simulink model "FlightGear_PID_try"  (R2017a)
settings: Solver=VariableStepAuto  StartTime=0.0  StopTime=20  RelTol=1e-3
values from neighbouring files (symbols this model uses):
  Fext_N = -g_EN * m    [HW5_4_surfaces.m]    (also in TEST_aerosetup.m = [10 10 10]; surfaces_setup_test.m)
  g_EN = [0; 0; 9.81]    [HW5_4_surfaces.m]    (also in TEST_aerosetup.m = [0; 0; 9.8]; surfaces_setup_test.m)
  J_cg = ones(3)    [HW5_4_surfaces.m]    (also in TEST_aerosetup.m)
  M_total = sum(MnG(:,1))/1000    [HW5_4_surfaces.m]    (also in TEST_aerosetup.m; surfaces_setup_test.m = sum(MnG1(:,1))/1000)
  Mext_B = [0; 0; 0]    [HW5_4_surfaces.m]    (also in TEST_aerosetup.m = [1; 1; 1]; surfaces_setup_test.m)
  p_E_BE_ini = p_E_BE_ini_deg .* [deg2rad; deg2rad; 1]    [HW5_4_surfaces.m]    (also in TEST_aerosetup.m; surfaces_setup_test.m)
  Rearth = 6371000    [HW5_4_surfaces.m]    (also in TEST_aerosetup.m; surfaces_setup_test.m)
  Theta_ini = Theta_ini_deg * deg2rad    [HW5_4_surfaces.m]    (also in TEST_aerosetup.m; surfaces_setup_test.m)
  v_N_AE = [0;0;0]    [HW5_4_surfaces.m]    (also in TEST_aerosetup.m; surfaces_setup_test.m)
  Vbbe_int = [10; 0; 0]    [HW5_4_surfaces.m]    (also in TEST_aerosetup.m; surfaces_setup_test.m = [5; 0; 0])
  w_B_BE_ini = [1e0; 1e-2; 1e-2]    [HW5_4_surfaces.m]    (also in TEST_aerosetup.m; surfaces_setup_test.m)
undefined symbols (not defined in the file or in its folder): Earth, WGS84
libraries: simulink x4, dspinverses x3, aerolibfltsims x2, vrlib x2, sharedtransform x1, aerolibtransform2 x1
settings Model: Creator=Jiaoran Wang  LastModifiedBy=Jiaoran Wang

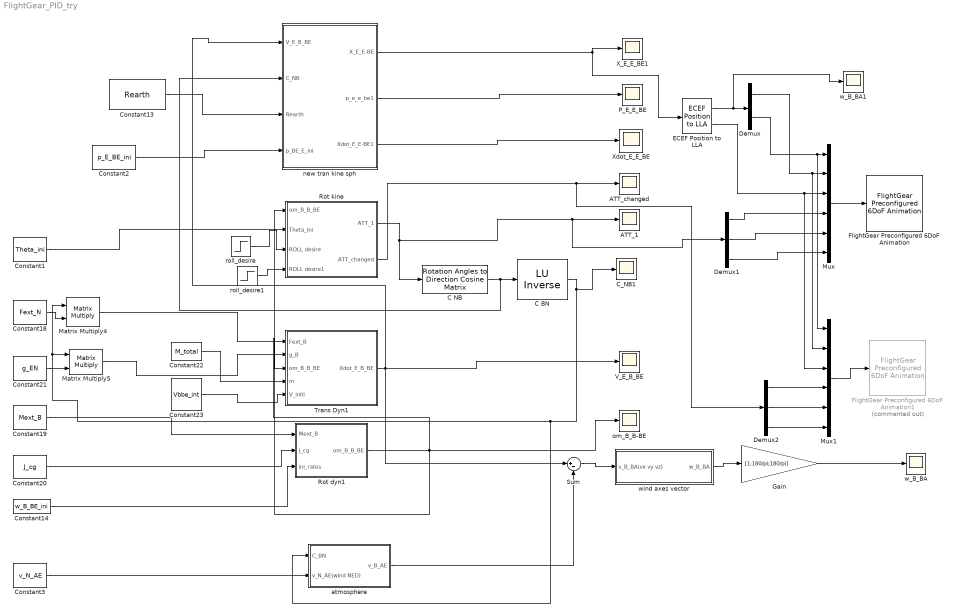
== system FlightGear_PID_try ==
  ATT_1 : Scope
  ATT_changed : Scope
  C BN : dspinverses/ LU Inverse
      settings: SourceProductName=DSP System Toolbox
  C NB : sharedtransform/Rotation Angles to Direction Cosine Matrix  rotationOrder=ZYX
  C_NB1 : Scope
  Constant1 : Constant  Value=Theta_ini
  Constant13 : Constant  Value=Rearth
  Constant14 : Constant  Value=w_B_BE_ini
  Constant18 : Constant  Value=Fext_N
  Constant19 : Constant  Value=Mext_B
  Constant2 : Constant  Value=p_E_BE_ini  VectorParams1D=off
  Constant20 : Constant  Value=J_cg
  Constant21 : Constant  Value=g_EN
  Constant22 : Constant  Value=M_total
  Constant23 : Constant  Value=Vbbe_int
  Constant3 : Constant  Value=v_N_AE
  Demux : Demux  Outputs=2
  Demux1 : Demux  Outputs=3
  Demux2 : Demux  Outputs=3
  ECEF Position to LLA : aerolibtransform2/ECEF Position to LLA  units=Metric (MKS)  ptype=Earth (WGS84)  F=1/298.257223563  R=6378137
      settings: SourceProductName=Aerospace Blockset  SourceProductBaseCode=AE
  FlightGear Preconfigured 6DoF Animation : aerolibfltsims/FlightGear Preconfigured 6DoF Animation  xFlightGearVersion=v3.0  DestinationIpAddress=127.0.0.1  DestinationPort=5502  SampleTime=1/50
      settings: SourceProductName=Aerospace Blockset
  FlightGear Preconfigured 6DoF Animation1 : aerolibfltsims/FlightGear Preconfigured 6DoF Animation  Commented=on  xFlightGearVersion=v3.0  DestinationIpAddress=127.0.0.1  DestinationPort=5502  SampleTime=1/50
      settings: SourceProductName=Aerospace Blockset
  Gain : Gain  Gain=[1;180/pi;180/pi]
  Matrix Multiply4 : Product  Multiplication=Matrix(*)
  Matrix Multiply5 : Product  Multiplication=Matrix(*)
  Mux : Mux  Inputs=6
  Mux1 : Mux  Inputs=6
  P_E_E_BE : Scope
  Rot dyn1 : Subsystem
  Rot kine : Subsystem
  Sum : Sum  Inputs=|+-
  Trans Dyn1 : Subsystem
  V_E_B_BE : Scope
  "X_E_E_BE1 " : Scope
  Xdot_E_E_BE : Scope
  atmosphere : Subsystem
  new tran kine sph : Subsystem
  om_B_B-BE : Scope
  roll_desire : Step  Time=0  After=0  SampleTime=0
  roll_desire1 : Step  Time=0  After=0  SampleTime=0
  w_B_BA : Scope
  w_B_BA1 : Scope
  wind axes vector : Subsystem
  wires:
  ECEF Position to LLA/1 -> w_B_BA1/1, Demux/1
  Constant2/1 -> new tran kine sph/4(p_BE_E_ini)
  Constant13/1 -> new tran kine sph/3(Rearth)
  C BN/1 -> C_NB1/1, atmosphere/1(C_BN), Matrix Multiply5/1, Matrix Multiply4/1
  Matrix Multiply5/1 -> Trans Dyn1/2(g_B)
  Demux/1 -> Mux1/2, Mux/2
  new tran kine sph/2(p_e_e_be1) -> P_E_E_BE/1
  Constant23/1 -> Trans Dyn1/5(V_initi)
  Matrix Multiply4/1 -> Trans Dyn1/1(Fext_B)
  Demux1/2 -> Mux/5
  ECEF Position to LLA/2 -> Mux1/3, Mux/3
  Constant18/1 -> Matrix Multiply4/2
  wind axes vector/1(w_B_BA) -> Gain/1
  atmosphere/1(v_B_AE) -> Sum/2
  Demux/2 -> Mux1/1, Mux/1
  Constant19/1 -> Rot dyn1/1(Mext_B)
  Constant3/1 -> atmosphere/2(v_N_AE(wind NED))
  new tran kine sph/1(X_E_E-BE) -> "X_E_E_BE1 "/1, ECEF Position to LLA/1
  new tran kine sph/3(Xdot_E_E-BE1) -> Xdot_E_E_BE/1
  Rot dyn1/1(om_B_B_BE) -> Rot kine/1(om_B_B_BE), om_B_B-BE/1, Trans Dyn1/3(om_B_B_BE)
  Constant14/1 -> Rot dyn1/3(ini_rates)
  Constant1/1 -> Rot kine/2(Theta_ini)
  Trans Dyn1/1(Xdot_E_B_BE) -> V_E_B_BE/1, Sum/1, new tran kine sph/1(V_E_B_BE)
  Constant22/1 -> Trans Dyn1/4(m)
  Constant21/1 -> Matrix Multiply5/2
  C NB/1 -> new tran kine sph/2(C_NB), C BN/1
  Sum/1 -> wind axes vector/1(v_B_BA(vx vy vz))
  Rot kine/1(ATT_1) -> Demux1/1, ATT_1/1, C NB/1
  Constant20/1 -> Rot dyn1/2(J_cg)
  Demux1/1 -> Mux/4
  Mux/1 -> FlightGear Preconfigured 6DoF Animation/1
  Gain/1 -> w_B_BA/1
  Demux1/3 -> Mux/6
  Rot kine/2(ATT_changed) -> Demux2/1, ATT_changed/1
  roll_desire/1 -> Rot kine/3(ROLL desire)
  roll_desire1/1 -> Rot kine/4(ROLL desire1)
  Mux1/1 -> FlightGear Preconfigured 6DoF Animation1/1
  Demux2/3 -> Mux1/6
  Demux2/2 -> Mux1/5
  Demux2/1 -> Mux1/4

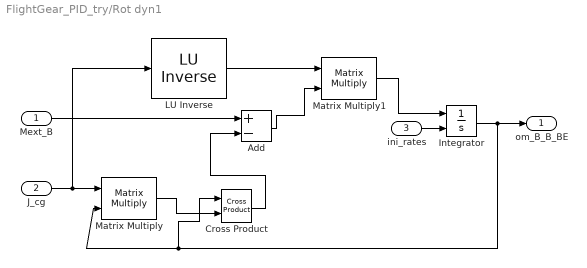
== system FlightGear_PID_try/Rot dyn1 ==
  Mext_B : Inport
  J_cg : Inport  Port=2
  ini_rates : Inport  Port=3
  " LU Inverse" : dspinverses/ LU Inverse
      settings: SourceProductName=DSP System Toolbox
  Add : Sum  Inputs=+-
  Cross Product : vrlib/Utilities/Cross Product
      settings: SourceProductBaseCode=VR
  Integrator : Integrator  InitialConditionSource=external
  Matrix Multiply : Product  Multiplication=Matrix(*)
  Matrix Multiply1 : Product  Multiplication=Matrix(*)
  om_B_B_BE : Outport
  wires:
  Mext_B/1 -> Add/1
  J_cg/1 -> " LU Inverse"/1, Matrix Multiply/1
  Matrix Multiply/1 -> Cross Product/2
  " LU Inverse"/1 -> Matrix Multiply1/1
  Add/1 -> Matrix Multiply1/2
  Cross Product/1 -> Add/2
  Matrix Multiply1/1 -> Integrator/1
  ini_rates/1 -> Integrator/2
  Integrator/1 -> Cross Product/1, Matrix Multiply/2, om_B_B_BE/1

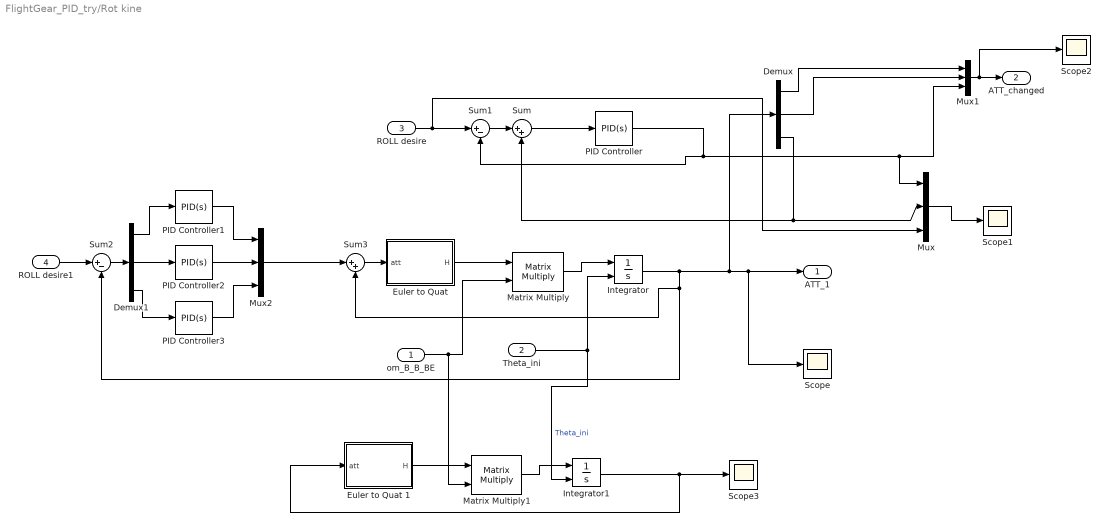
== system FlightGear_PID_try/Rot kine ==
  om_B_B_BE : Inport
  Theta_ini : Inport  Port=2
  ROLL desire : Inport  Port=3
  ROLL desire1 : Inport  Port=4
  Demux : Demux  Outputs=3
  Demux1 : Demux  Outputs=3
  "Euler to Quat " : MATLAB Function  TreatAsAtomicUnit=on
  Euler to Quat 1 : MATLAB Function  TreatAsAtomicUnit=on
  Integrator : Integrator  InitialConditionSource=external
  Integrator1 : Integrator  InitialConditionSource=external
  Matrix Multiply : Product  Multiplication=Matrix(*)
  Matrix Multiply1 : Product  Multiplication=Matrix(*)
  Mux : Mux  Inputs=3
  Mux1 : Mux  Inputs=3
  Mux2 : Mux  Inputs=3
  PID Controller : simulink/Continuous/PID Controller  Controller=PID  TimeDomain=Continuous-time  SampleTime=-1  IntegratorMethod=Forward Euler  FilterMethod=Forward Euler  Form=Parallel  UseFilter=on  ControllerParametersSource=internal  P=0  I=10  D=0  N=100  InitialConditionSource=internal  InitialConditionForIntegrator=0  InitialConditionForFilter=0  ExternalReset=none  LimitOutput=off  UpperSaturationLimit=inf  LowerSaturationLimit=-inf  LinearizeAsGain=on  AntiWindupMode=none  Kb=1  TrackingMode=off  Kt=1  PParamMin=[]  PParamMax=[]  IParamMin=[]  IParamMax=[]  DParamMin=[]  DParamMax=[]  NParamMin=[]  NParamMax=[]  KbParamMin=[]  KbParamMax=[]  KtParamMin=[]  KtParamMax=[]  POutMin=[]  POutMax=[]  IOutMin=[]  IOutMax=[]  DOutMin=[]  DOutMax=[]  NOutMin=[]  NOutMax=[]  KbOutMin=[]  KbOutMax=[]  KtOutMin=[]  KtOutMax=[]  IntegratorOutMin=[]  IntegratorOutMax=[]  FilterOutMin=[]  FilterOutMax=[]  SumOutMin=[]  SumOutMax=[]  SumI1OutMin=[]  SumI1OutMax=[]  SumI2OutMin=[]  SumI2OutMax=[]  SumI3OutMin=[]  SumI3OutMax=[]  SumDOutMin=[]  SumDOutMax=[]  SaturationOutMin=[]  SaturationOutMax=[]  IntegratorContinuousStateAttributes=''  IntegratorStateMustResolveToSignalObject=off  IntegratorRTWStateStorageClass=Auto  FilterContinuousStateAttributes=''  FilterStateMustResolveToSignalObject=off  FilterRTWStateStorageClass=Auto  DifferentiatorICPrevScaledInput=0  DifferentiatorOutMin=[]  DifferentiatorOutMax=[]  InitialConditionSetting=State (most efficient)
  PID Controller1 : simulink/Continuous/PID Controller  Controller=PID  TimeDomain=Continuous-time  SampleTime=-1  IntegratorMethod=Forward Euler  FilterMethod=Forward Euler  Form=Parallel  UseFilter=on  ControllerParametersSource=internal  P=0  I=10  D=1  N=100  InitialConditionSource=internal  InitialConditionForIntegrator=0  InitialConditionForFilter=0  ExternalReset=none  LimitOutput=off  UpperSaturationLimit=inf  LowerSaturationLimit=-inf  LinearizeAsGain=on  AntiWindupMode=none  Kb=1  TrackingMode=off  Kt=1  PParamMin=[]  PParamMax=[]  IParamMin=[]  IParamMax=[]  DParamMin=[]  DParamMax=[]  NParamMin=[]  NParamMax=[]  KbParamMin=[]  KbParamMax=[]  KtParamMin=[]  KtParamMax=[]  POutMin=[]  POutMax=[]  IOutMin=[]  IOutMax=[]  DOutMin=[]  DOutMax=[]  NOutMin=[]  NOutMax=[]  KbOutMin=[]  KbOutMax=[]  KtOutMin=[]  KtOutMax=[]  IntegratorOutMin=[]  IntegratorOutMax=[]  FilterOutMin=[]  FilterOutMax=[]  SumOutMin=[]  SumOutMax=[]  SumI1OutMin=[]  SumI1OutMax=[]  SumI2OutMin=[]  SumI2OutMax=[]  SumI3OutMin=[]  SumI3OutMax=[]  SumDOutMin=[]  SumDOutMax=[]  SaturationOutMin=[]  SaturationOutMax=[]  IntegratorContinuousStateAttributes=''  IntegratorStateMustResolveToSignalObject=off  IntegratorRTWStateStorageClass=Auto  FilterContinuousStateAttributes=''  FilterStateMustResolveToSignalObject=off  FilterRTWStateStorageClass=Auto  DifferentiatorICPrevScaledInput=0  DifferentiatorOutMin=[]  DifferentiatorOutMax=[]  InitialConditionSetting=State (most efficient)
  PID Controller2 : simulink/Continuous/PID Controller  Controller=PID  TimeDomain=Continuous-time  SampleTime=-1  IntegratorMethod=Forward Euler  FilterMethod=Forward Euler  Form=Parallel  UseFilter=on  ControllerParametersSource=internal  P=0  I=10  D=0  N=100  InitialConditionSource=internal  InitialConditionForIntegrator=0  InitialConditionForFilter=0  ExternalReset=none  LimitOutput=off  UpperSaturationLimit=inf  LowerSaturationLimit=-inf  LinearizeAsGain=on  AntiWindupMode=none  Kb=1  TrackingMode=off  Kt=1  PParamMin=[]  PParamMax=[]  IParamMin=[]  IParamMax=[]  DParamMin=[]  DParamMax=[]  NParamMin=[]  NParamMax=[]  KbParamMin=[]  KbParamMax=[]  KtParamMin=[]  KtParamMax=[]  POutMin=[]  POutMax=[]  IOutMin=[]  IOutMax=[]  DOutMin=[]  DOutMax=[]  NOutMin=[]  NOutMax=[]  KbOutMin=[]  KbOutMax=[]  KtOutMin=[]  KtOutMax=[]  IntegratorOutMin=[]  IntegratorOutMax=[]  FilterOutMin=[]  FilterOutMax=[]  SumOutMin=[]  SumOutMax=[]  SumI1OutMin=[]  SumI1OutMax=[]  SumI2OutMin=[]  SumI2OutMax=[]  SumI3OutMin=[]  SumI3OutMax=[]  SumDOutMin=[]  SumDOutMax=[]  SaturationOutMin=[]  SaturationOutMax=[]  IntegratorContinuousStateAttributes=''  IntegratorStateMustResolveToSignalObject=off  IntegratorRTWStateStorageClass=Auto  FilterContinuousStateAttributes=''  FilterStateMustResolveToSignalObject=off  FilterRTWStateStorageClass=Auto  DifferentiatorICPrevScaledInput=0  DifferentiatorOutMin=[]  DifferentiatorOutMax=[]  InitialConditionSetting=State (most efficient)
  PID Controller3 : simulink/Continuous/PID Controller  Controller=PID  TimeDomain=Continuous-time  SampleTime=-1  IntegratorMethod=Forward Euler  FilterMethod=Forward Euler  Form=Parallel  UseFilter=on  ControllerParametersSource=internal  P=0  I=10  D=0  N=100  InitialConditionSource=internal  InitialConditionForIntegrator=0  InitialConditionForFilter=0  ExternalReset=none  LimitOutput=off  UpperSaturationLimit=inf  LowerSaturationLimit=-inf  LinearizeAsGain=on  AntiWindupMode=none  Kb=1  TrackingMode=off  Kt=1  PParamMin=[]  PParamMax=[]  IParamMin=[]  IParamMax=[]  DParamMin=[]  DParamMax=[]  NParamMin=[]  NParamMax=[]  KbParamMin=[]  KbParamMax=[]  KtParamMin=[]  KtParamMax=[]  POutMin=[]  POutMax=[]  IOutMin=[]  IOutMax=[]  DOutMin=[]  DOutMax=[]  NOutMin=[]  NOutMax=[]  KbOutMin=[]  KbOutMax=[]  KtOutMin=[]  KtOutMax=[]  IntegratorOutMin=[]  IntegratorOutMax=[]  FilterOutMin=[]  FilterOutMax=[]  SumOutMin=[]  SumOutMax=[]  SumI1OutMin=[]  SumI1OutMax=[]  SumI2OutMin=[]  SumI2OutMax=[]  SumI3OutMin=[]  SumI3OutMax=[]  SumDOutMin=[]  SumDOutMax=[]  SaturationOutMin=[]  SaturationOutMax=[]  IntegratorContinuousStateAttributes=''  IntegratorStateMustResolveToSignalObject=off  IntegratorRTWStateStorageClass=Auto  FilterContinuousStateAttributes=''  FilterStateMustResolveToSignalObject=off  FilterRTWStateStorageClass=Auto  DifferentiatorICPrevScaledInput=0  DifferentiatorOutMin=[]  DifferentiatorOutMax=[]  InitialConditionSetting=State (most efficient)
  Scope{,1..3} (4 alike) : Scope
  Sum : Sum  Inputs=|++
  Sum1 : Sum  Inputs=|+-
  Sum2 : Sum  Inputs=|+-
  Sum3 : Sum  Inputs=|++
  ATT_1 : Outport
  ATT_changed : Outport  Port=2
  wires:
  om_B_B_BE/1 -> Matrix Multiply1/2, Matrix Multiply/2
  Integrator/1 -> Sum3/2, Sum2/2, Scope/1, ATT_1/1, Demux/1
  "Euler to Quat "/1(H) -> Matrix Multiply/1
  Theta_ini/1 -> Integrator/2, Integrator1/2  "Theta_ini"
  Matrix Multiply/1 -> Integrator/1
  Demux/3 -> Sum/2, Mux/2
  Demux/1 -> Mux1/1
  PID Controller/1 -> Sum1/2, Mux/1, Mux1/3
  Mux/1 -> Scope1/1
  Demux/2 -> Mux1/2
  Mux1/1 -> Scope2/1, ATT_changed/1
  ROLL desire/1 -> Sum1/1, Mux/3
  Sum1/1 -> Sum/1
  Sum/1 -> PID Controller/1
  ROLL desire1/1 -> Sum2/1
  Sum3/1 -> "Euler to Quat "/1(att)
  Matrix Multiply1/1 -> Integrator1/1
  Euler to Quat 1/1(H) -> Matrix Multiply1/1
  Demux1/1 -> PID Controller1/1
  Sum2/1 -> Demux1/1
  Demux1/2 -> PID Controller2/1
  Demux1/3 -> PID Controller3/1
  Mux2/1 -> Sum3/1
  PID Controller1/1 -> Mux2/1
  PID Controller2/1 -> Mux2/2
  PID Controller3/1 -> Mux2/3
  Integrator1/1 -> Euler to Quat 1/1(att), Scope3/1

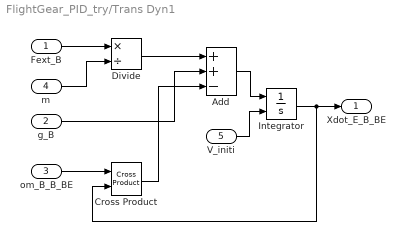
== system FlightGear_PID_try/Trans Dyn1 ==
  Fext_B : Inport
  g_B : Inport  Port=2
  om_B_B_BE : Inport  Port=3
  m : Inport  Port=4
  V_initi : Inport  Port=5
  Add : Sum  Inputs=++-
  Cross Product : vrlib/Utilities/Cross Product
      settings: SourceProductBaseCode=VR
  Divide : Product  Inputs=*/
  Integrator : Integrator  InitialConditionSource=external
  Xdot_E_B_BE : Outport
  wires:
  Fext_B/1 -> Divide/1
  m/1 -> Divide/2
  Divide/1 -> Add/1
  g_B/1 -> Add/2
  om_B_B_BE/1 -> Cross Product/1
  Cross Product/1 -> Add/3
  Add/1 -> Integrator/1
  V_initi/1 -> Integrator/2
  Integrator/1 -> Cross Product/2, Xdot_E_B_BE/1

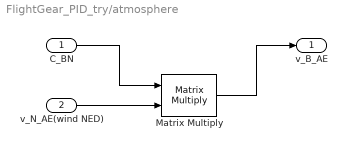
== system FlightGear_PID_try/atmosphere ==
  C_BN : Inport
  v_N_AE(wind NED) : Inport  Port=2
  Matrix Multiply : Product  Multiplication=Matrix(*)
  v_B_AE : Outport
  wires:
  v_N_AE(wind NED)/1 -> Matrix Multiply/2
  C_BN/1 -> Matrix Multiply/1
  Matrix Multiply/1 -> v_B_AE/1

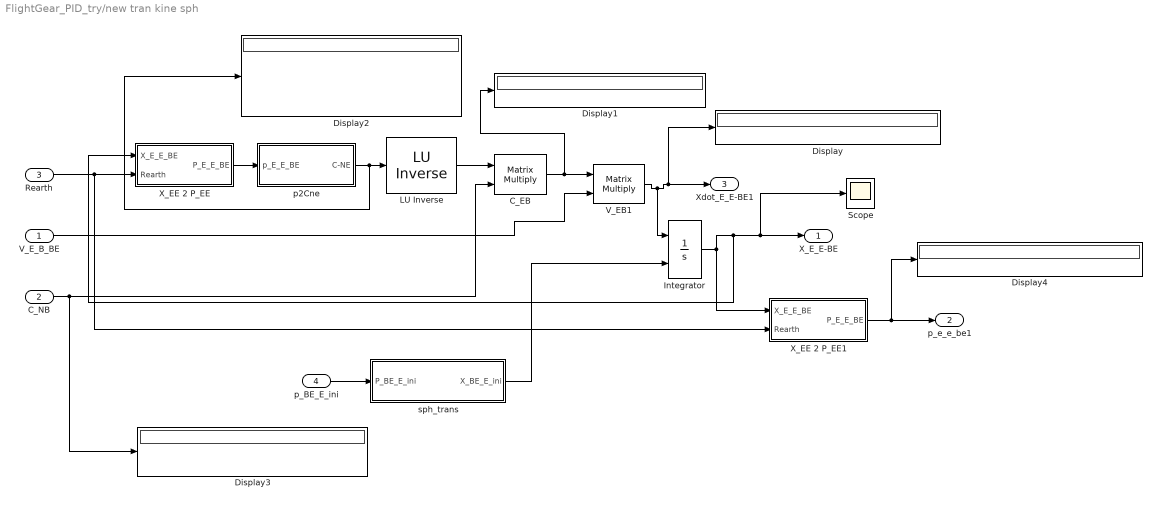
== system FlightGear_PID_try/new tran kine sph ==
  V_E_B_BE : Inport
  C_NB : Inport  Port=2
  Rearth : Inport  Port=3
  p_BE_E_ini : Inport  Port=4
  " LU Inverse" : dspinverses/ LU Inverse
      settings: SourceProductName=DSP System Toolbox
  C_EB : Product  Multiplication=Matrix(*)
  Display{,1..4} (5 alike) : Display
  Integrator : Integrator  InitialConditionSource=external
  Scope : Scope
  V_EB1 : Product  Multiplication=Matrix(*)
  X_EE 2 P_EE : Subsystem
  X_EE 2 P_EE1 : Subsystem
  p2Cne : Subsystem
  sph_trans : MATLAB Function  TreatAsAtomicUnit=on
  X_E_E-BE : Outport
  p_e_e_be1 : Outport  Port=2
  Xdot_E_E-BE1 : Outport  Port=3
  wires:
  " LU Inverse"/1 -> C_EB/1
  Integrator/1 -> Scope/1, X_E_E-BE/1, X_EE 2 P_EE/1(X_E_E_BE), X_EE 2 P_EE1/1(X_E_E_BE)
  X_EE 2 P_EE1/1(P_E_E_BE) -> Display4/1, p_e_e_be1/1
  Rearth/1 -> X_EE 2 P_EE1/2(Rearth), X_EE 2 P_EE/2(Rearth)
  V_EB1/1 -> Display/1, Xdot_E_E-BE1/1, Integrator/1
  C_EB/1 -> Display1/1, V_EB1/1
  p2Cne/1(C-NE) -> Display2/1, " LU Inverse"/1
  X_EE 2 P_EE/1(P_E_E_BE) -> p2Cne/1(p_E_E_BE)
  C_NB/1 -> Display3/1, C_EB/2
  V_E_B_BE/1 -> V_EB1/2
  p_BE_E_ini/1 -> sph_trans/1(P_BE_E_ini)
  sph_trans/1(X_BE_E_ini) -> Integrator/2

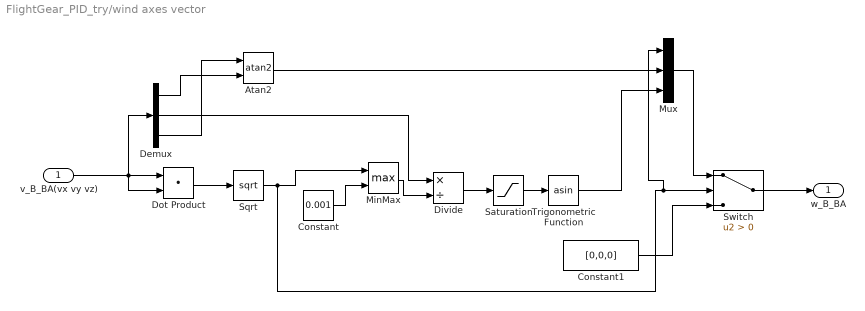
== system FlightGear_PID_try/wind axes vector ==
  v_B_BA(vx vy vz) : Inport
  Atan2 : Trigonometry  Operator=atan2
  Constant : Constant  Value=0.001
  Constant1 : Constant  Value=[0,0,0]
  Demux : Demux  Outputs=3
  Divide : Product  Inputs=*/
  Dot Product : DotProduct  InputSameDT=on  OutDataTypeStr=Inherit: Inherit via internal rule
  MinMax : MinMax  Function=max  Inputs=2
  Mux : Mux  Inputs=3
  Saturation : Saturate
  Sqrt : Sqrt  SaturateOnIntegerOverflow=on
  Switch : Switch  Criteria=u2 > Threshold
  Trigonometric Function : Trigonometry  Operator=asin  ApproximationMethod=CORDIC
  w_B_BA : Outport
  wires:
  v_B_BA(vx vy vz)/1 -> Demux/1, Dot Product/2, Dot Product/1
  Dot Product/1 -> Sqrt/1
  Sqrt/1 -> Mux/1, Switch/2, MinMax/1
  Constant/1 -> MinMax/2
  MinMax/1 -> Divide/2
  Demux/2 -> Divide/1
  Demux/3 -> Atan2/1
  Demux/1 -> Atan2/2
  Atan2/1 -> Mux/2
  Divide/1 -> Saturation/1
  Saturation/1 -> Trigonometric Function/1
  Trigonometric Function/1 -> Mux/3
  Constant1/1 -> Switch/3
  Mux/1 -> Switch/1
  Switch/1 -> w_B_BA/1

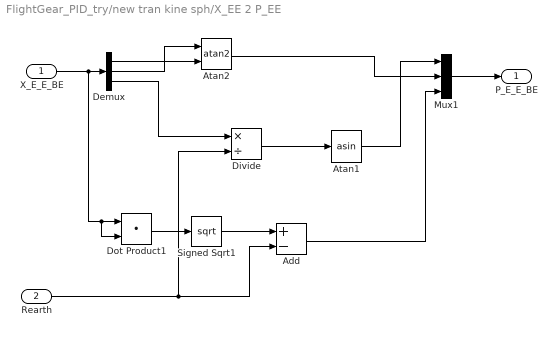
== system FlightGear_PID_try/new tran kine sph/X_EE 2 P_EE ==
  X_E_E_BE : Inport
  Rearth : Inport  Port=2
  Add : Sum  Inputs=+-
  Atan1 : Trigonometry  Operator=asin
  Atan2 : Trigonometry  Operator=atan2
  Demux : Demux  Outputs=3
  Divide : Product  Inputs=*/
  Dot Product1 : DotProduct  InputSameDT=on  OutDataTypeStr=Inherit: Inherit via internal rule
  Mux1 : Mux  Inputs=3
  Signed Sqrt1 : Sqrt  SaturateOnIntegerOverflow=on
  P_E_E_BE : Outport
  wires:
  X_E_E_BE/1 -> Dot Product1/2, Dot Product1/1, Demux/1
  Demux/1 -> Atan2/2
  Demux/2 -> Atan2/1
  Atan2/1 -> Mux1/2
  Dot Product1/1 -> Signed Sqrt1/1
  Signed Sqrt1/1 -> Add/1
  Rearth/1 -> Divide/2, Add/2
  Add/1 -> Mux1/3
  Mux1/1 -> P_E_E_BE/1
  Demux/3 -> Divide/1
  Divide/1 -> Atan1/1
  Atan1/1 -> Mux1/1

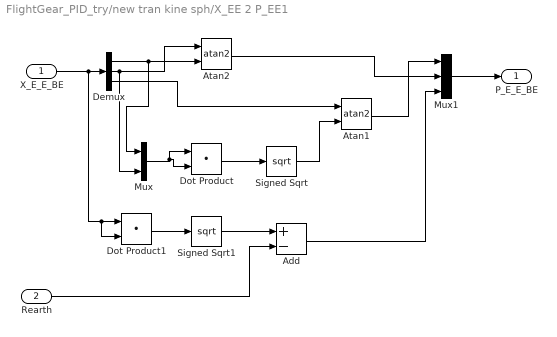
== system FlightGear_PID_try/new tran kine sph/X_EE 2 P_EE1 ==
  X_E_E_BE : Inport
  Rearth : Inport  Port=2
  Add : Sum  Inputs=+-
  Atan1 : Trigonometry  Operator=atan2
  Atan2 : Trigonometry  Operator=atan2
  Demux : Demux  Outputs=3
  Dot Product : DotProduct  InputSameDT=on  OutDataTypeStr=Inherit: Inherit via internal rule
  Dot Product1 : DotProduct  InputSameDT=on  OutDataTypeStr=Inherit: Inherit via internal rule
  Mux : Mux  Inputs=2
  Mux1 : Mux  Inputs=3
  Signed Sqrt : Sqrt  SaturateOnIntegerOverflow=on
  Signed Sqrt1 : Sqrt  SaturateOnIntegerOverflow=on
  P_E_E_BE : Outport
  wires:
  X_E_E_BE/1 -> Dot Product1/2, Dot Product1/1, Demux/1
  Demux/1 -> Mux/1, Atan2/2
  Demux/2 -> Atan2/1, Mux/2
  Mux/1 -> Dot Product/2, Dot Product/1
  Dot Product/1 -> Signed Sqrt/1
  Signed Sqrt/1 -> Atan1/2
  Demux/3 -> Atan1/1
  Atan2/1 -> Mux1/2
  Atan1/1 -> Mux1/1
  Dot Product1/1 -> Signed Sqrt1/1
  Signed Sqrt1/1 -> Add/1
  Rearth/1 -> Add/2
  Add/1 -> Mux1/3
  Mux1/1 -> P_E_E_BE/1

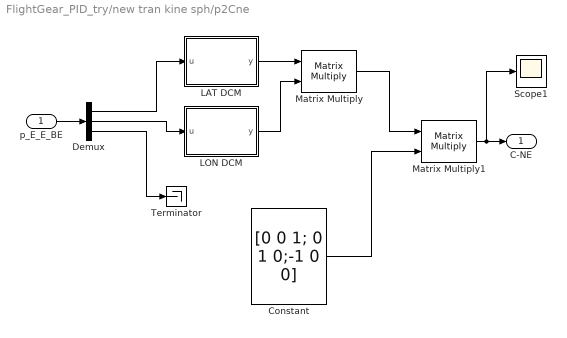
== system FlightGear_PID_try/new tran kine sph/p2Cne ==
  p_E_E_BE : Inport
  Constant : Constant  Value=[0 0 1; 0 1 0;-1 0 0]
  Demux : Demux  Outputs=3
  LAT DCM : MATLAB Function  TreatAsAtomicUnit=on
  LON DCM : MATLAB Function  TreatAsAtomicUnit=on
  Matrix Multiply : Product  Multiplication=Matrix(*)
  Matrix Multiply1 : Product  Multiplication=Matrix(*)
  Scope1 : Scope
  Terminator : Terminator
  C-NE : Outport
  wires:
  p_E_E_BE/1 -> Demux/1
  Demux/3 -> Terminator/1
  Demux/2 -> LON DCM/1(u)
  Demux/1 -> LAT DCM/1(u)
  LAT DCM/1(y) -> Matrix Multiply/1
  LON DCM/1(y) -> Matrix Multiply/2
  Matrix Multiply/1 -> Matrix Multiply1/1
  Constant/1 -> Matrix Multiply1/2
  Matrix Multiply1/1 -> Scope1/1, C-NE/1

== matlab function FlightGear_PID_try/new tran kine sph/p2Cne/LAT DCM ==
  data: u input; y output
function y = fcn(u)
y = [cos(u) 0 sin(u); 0 1 0; -sin(u) 0 cos(u)];

== matlab function FlightGear_PID_try/Rot kine/Euler to Quat 1 ==
  data: att input; H output
function H = fcn(att)
%#codegen
phi=att(1);
theta=att(2);
%psi=theta(3); %not needed for Euler Rotational Kinematics Matrix
H=[1,tan(theta)*sin(phi),tan(theta)*cos(phi); 0,cos(phi),-sin(phi);0,sin(phi)/cos(theta),cos(phi)/cos(theta)];

== matlab function FlightGear_PID_try/new tran kine sph/p2Cne/LON DCM ==
  data: u input; y output
function y = fcn(u)

y = [1, 0, 0;0, cos(u), sin(u);0, -sin(u), cos(u)];

== matlab function FlightGear_PID_try/Rot kine/Euler to Quat  ==
  data: att input; H output
function H = fcn(att)
%#codegen
phi=att(1);
theta=att(2);
%psi=theta(3); %not needed for Euler Rotational Kinematics Matrix
H=[1,tan(theta)*sin(phi),tan(theta)*cos(phi); 0,cos(phi),-sin(phi);0,sin(phi)/cos(theta),cos(phi)/cos(theta)];

== matlab function FlightGear_PID_try/new tran kine sph/sph_trans ==
  data: P_BE_E_ini input; X_BE_E_ini output
function X_BE_E_ini = fcn(P_BE_E_ini)
lat=P_BE_E_ini(1);
lon=P_BE_E_ini(2);
alt=P_BE_E_ini(3);
a = 6378000;
e = 8.1819190842622e-2;
N = a ./ sqrt(1 - e^2 .* sin(lat).^2);
x = (N+alt) .* cos(lat) .* cos(lon);
y = (N+alt) .* cos(lat) .* sin(lon);
z = ((1-e^2) .* N + alt) .* sin(lat);
X_BE_E_ini=[(N+alt) .* cos(lat) .* cos(lon); (N+alt) .* cos(lat) .* sin(lon);((1-e^2) .* N + alt) .* sin(lat)];
